simulink model "Baseband_LDPC_QPSK_CRC_MULTIPATH"  (R2017b)
settings: Solver=FixedStepDiscrete  StartTime=0.0  StopTime=20  RelTol=1e-3
undefined symbols (not defined in the file or in its folder): dvbs2ldpc
libraries: commdigbbndpm3 x4, commchan3 x2, commsink2 x2, commcrc2 x2, commblkcod2 x2, commdigbbndam3 x2, commrandsrc3 x1
settings Model: NumberOfSteps=3  Creator=m.s  LastModifiedBy=m.s

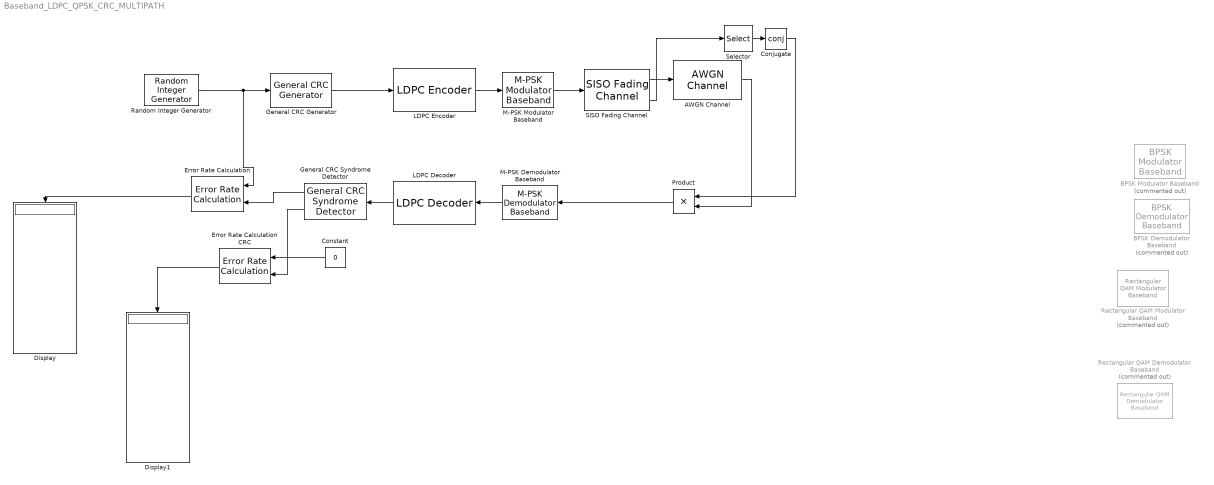
== system Baseband_LDPC_QPSK_CRC_MULTIPATH ==
  AWGN Channel : commchan3/AWGN Channel  InputProcessing=Columns as channels (frame based)  seed=67  noiseMode="Signal to noise ratio  (SNR)"  EbNodB=10  EsNodB=10  SNRdB=0  bitsPerSym=1  Ps=1  Tsym=1  variance=1
  BPSK Demodulator Baseband : commdigbbndpm3/BPSK Demodulator Baseband  Commented=on  DecType=Log-likelihood ratio  VarSource=Dialog  Variance=1  Ph=0  outDtype=Inherit via internal rule  derotateFactorWordLen=16  derotateFactorDataTypeStr=Inherit: Same word length as input  derotateFactorLastDataTypeStr=Inherit: Same word length as input
  BPSK Modulator Baseband : commdigbbndpm3/BPSK Modulator Baseband  Commented=on  Ph=0  outDtype=double  outWordLen=16  outUDDataType=sfix(16)  outFracLenMode=Best precision  outFracLen=15  outDataTypeStr=double  outLastDataTypeStr=double
  Conjugate : Math  Operator=conj  RndMeth=Zero  SaturateOnIntegerOverflow=on
  Constant : Constant  Value=0
  Display : Display
  Display1 : Display
  Error Rate Calculation : commsink2/Error Rate Calculation  N=0  st_delay=0  cp_mode=Entire frame  subframe=[]  PMode=Port  WsName=ErrorVec  RsMode2=off  stop=off  numErr=100  maxBits=1e6
  Error Rate Calculation CRC : commsink2/Error Rate Calculation  N=0  st_delay=0  cp_mode=Entire frame  subframe=[]  PMode=Port  WsName=ErrorVec  RsMode2=off  stop=off  numErr=100  maxBits=1e6
  General CRC Generator : commcrc2/General CRC Generator  genPoly=[16 12 5 0]  iniStates=0  directMethod=on  reflectInputBytes=off  reflectChecksums=off  finalXOR=0  numChecksums=1
      settings: SourceProductName=Communications System Toolbox  SourceProductBaseCode=CM
  General CRC Syndrome Detector : commcrc2/General CRC Syndrome Detector  genPoly=[16 12 5 0]  iniStates=0  directMethod=on  reflectInputBytes=off  reflectChecksums=off  finalXOR=0  numChecksums=1
      settings: SourceProductName=Communications System Toolbox  SourceProductBaseCode=CM
  LDPC Decoder : commblkcod2/LDPC Decoder  ParityCheckMat=dvbs2ldpc(1/2)  OutputFmt=Information part  DecisionType=Soft decision  OutputDataType=double  NumIter=50  DoParityCheck=off  OutputNumIter=off  OutputFinalChecks=off
      settings: SourceProductName=Communications System Toolbox  SourceProductBaseCode=CM
  LDPC Encoder : commblkcod2/LDPC Encoder  ParityCheckMat=dvbs2ldpc(1/2)
      settings: SourceProductName=Communications System Toolbox  SourceProductBaseCode=CM
  M-PSK Demodulator Baseband : commdigbbndpm3/M-PSK Demodulator Baseband  M=4  OutType=Bit  DecType=Hard decision  VarSource=Dialog  Variance=0.001  Dec=Gray  Mapping=[0:7]  Ph=pi/4  outDtype1=double  outDtype2=Inherit via internal rule  derotateFactorWordLen=16  derotateFactorDataTypeStr=Inherit: Same word length as input  derotateFactorLastDataTypeStr=Inherit: Same word length as input
      settings: SourceProductName=Communications System Toolbox
  M-PSK Modulator Baseband : commdigbbndpm3/M-PSK Modulator Baseband  M=4  InType=Bit  Enc=Gray  Mapping=[0:7]  Ph=pi/4  outDtype=double  outWordLen=16  outUDDataType=sfix(16)  outFracLenMode=Best precision  outFracLen=15  outDataTypeStr=double  outLastDataTypeStr=double
      settings: SourceProductName=Communications System Toolbox
  Product : Product
  Random Integer Generator : commrandsrc3/Random Integer Generator  SetSize=2  SeedSource=Parameter  Seed=0  SampleTime=1e-4  SamplesPerFrame=32384  OutputDataType=double  SimulateUsing=Interpreted execution
  Rectangular QAM Demodulator Baseband : commdigbbndam3/Rectangular QAM Demodulator Baseband  Commented=on  M=16  OutType=Bit  DecType=Log-likelihood ratio  VarSource=Dialog  Variance=1  Dec=Gray  Mapping=[0:15]  PowType=Average Power  MinDist=2  AvgPow=1  PeakPow=1  Ph=0  outDtype1=Inherit via internal rule  outDtype2=Inherit via internal rule  derotateFactorWordLen=16  derotateFactorDataTypeStr=Inherit: Same word length as input  derotateFactorLastDataTypeStr=Inherit: Same word length as input  denormFactorWordLen=16  denormFactorDataTypeStr=Inherit: Same word length as input  denormFactorLastDataTypeStr=Inherit: Same word length as input  prodOutWordLen=32  prodOutOverflowMode=Wrap  prodOutRoundingMode=Floor  prodOutOvFlMode=off  prodOutOvFlModeLastStrValue=off  sumWordLen=32
  Rectangular QAM Modulator Baseband : commdigbbndam3/Rectangular QAM Modulator Baseband  Commented=on  M=16  InType=Bit  Enc=Gray  Mapping=[0:15]  PowType=Average Power  MinDist=2  AvgPow=1  PeakPow=1  Ph=0  outDtype=double  outWordLen=16  outUDDataType=sfix(16)  outFracLenMode=Best precision  outFracLen=15  outDataTypeStr=double  outLastDataTypeStr=double
  SISO Fading Channel : commchan3/SISO Fading Channel  PathDelays=[0 1e-4 2e-4]  AveragePathGains=[0 -6 -12]  NormalizePathGains=on  FadingDistribution=Rayleigh  KFactor=3  DirectPathDopplerShift=0  DirectPathInitialPhase=0  MaximumDopplerShift=30  DopplerSpectrum=ds  RandomStream=mt19937ar with seed  RandomNumGenerator=mt19937ar  Seed=73  PathGainsOutputPort=on  ChannelFilterDelayOutputPort=off  SimulateUsing=Interpreted execution  Visualization=Off  PathsForDopplerDisplay=1  SamplesToDisplay=25%
      settings: SourceProductName=Communications System Toolbox
  Selector : Selector  NumberOfDimensions=2  InputPortWidth=3  IndexOptions=Select all,Index vector (dialog)  Indices=1,1  OutputSizes=1,1
  wires:
  Error Rate Calculation/1 -> Display/1
  Random Integer Generator/1 -> Error Rate Calculation/1, General CRC Generator/1
  SISO Fading Channel/2 -> Selector/1
  Selector/1 -> Conjugate/1
  Conjugate/1 -> Product/1
  LDPC Encoder/1 -> M-PSK Modulator Baseband/1
  M-PSK Demodulator Baseband/1 -> LDPC Decoder/1
  SISO Fading Channel/1 -> AWGN Channel/1
  AWGN Channel/1 -> Product/2
  Constant/1 -> Error Rate Calculation CRC/1
  General CRC Generator/1 -> LDPC Encoder/1
  LDPC Decoder/1 -> General CRC Syndrome Detector/1
  General CRC Syndrome Detector/1 -> Error Rate Calculation/2
  General CRC Syndrome Detector/2 -> Error Rate Calculation CRC/2
  Error Rate Calculation CRC/1 -> Display1/1
  Product/1 -> M-PSK Demodulator Baseband/1
  M-PSK Modulator Baseband/1 -> SISO Fading Channel/1
